simulink model "PID_mgtXY_loadingTest_video"  (R2023a)
settings: Solver=VariableStepAuto  StartTime=0.0  StopTime=t_sim/10  RelTol=1e-3
undefined symbols (not defined in the file or in its folder): A, B, DeltaH_error_Gain, Error_ref_Gain, I, J, juliandate, Ke, Kt, La, magnetic_field, Mgt_power_Gain, n_cal, omegaZ_inicial, R_mgt, Ra, RW_omega_max, RW_power_Gain, T_ext, T_max, T_max_mgt, yaw_ref
libraries: slpidlib x12, matrix_library x10, simulink_extras x6, sharedutil x3, simulink x2, vrlib x2, aerolibutil x1, sharedtransform x1, aerolibcubesatveh x1, aerolibgravity2 x1
(part 1 of 2)
settings Model: Creator=Personal  LastModifiedBy=Personal
settings SolverCC: ZeroCrossAlgorithm=Adaptive
settings DebuggingCC: IgnoredZcDiagnostic=none

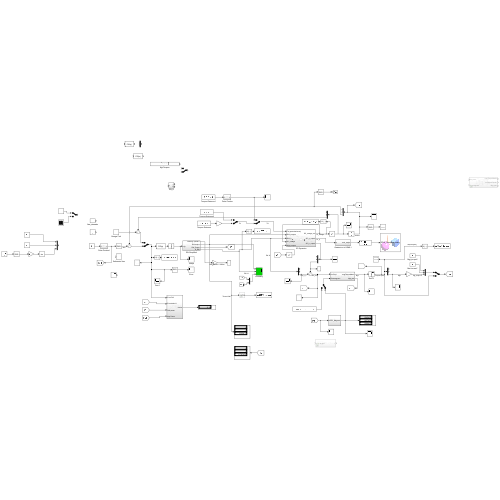
[thumbnail: Simulink's stored preview of the top-level diagram]
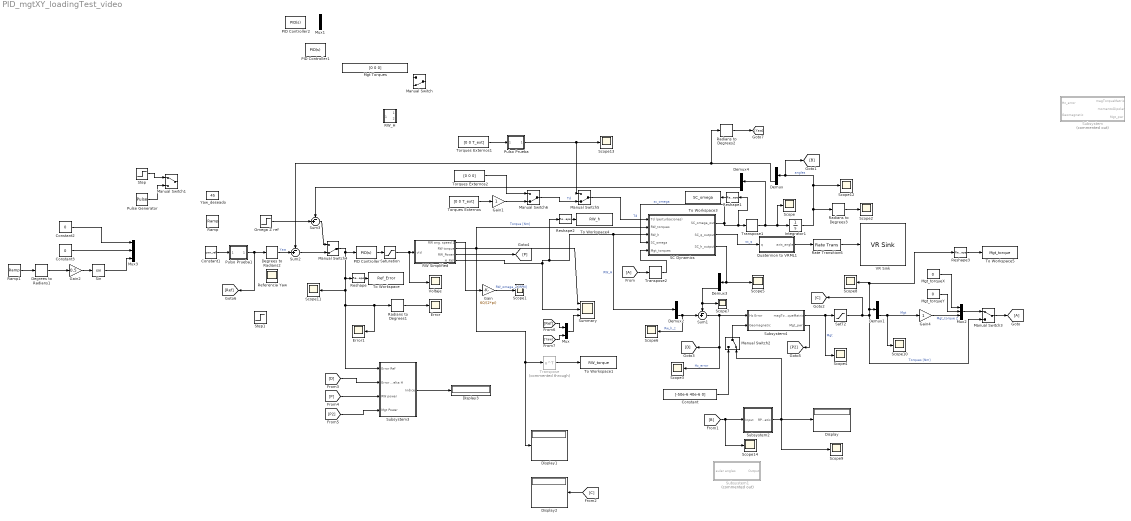
== system PID_mgtXY_loadingTest_video ==
  Constant : Constant  Value=[-50e-6 40e-6 0]
  Constant1 : Constant  Value=yaw_ref
  Constant2 : Constant  Value=0
  Constant3 : Constant  Value=0
  Degrees to Radians1 : simulink_extras/Transformations/Degrees to Radians
  Degrees to Radians2 : simulink_extras/Transformations/Degrees to Radians
  Demux{,1..4} (5 alike) : Demux  Outputs=3
  Display{,1..3} (4 alike) : Display
  Error : Scope
  Error1 : Scope
  From : From
  Gain : Gain  Gain=60/(2*pi)
  Gain1 : Gain
  Gain2 : Gain  Gain=0.5
  Gain4 : Gain
  Goto : Goto
  Integrator1 : Integrator  InitialCondition=[0 0 0]
  Manual Switch{,2,4..6} (5 alike) : ManualSwitch  CurrentSetting=0
  Manual Switch1 : ManualSwitch
  Manual Switch3 : ManualSwitch
  Mgt Torques : Constant  Value=[0 0 0]
  Mgt_torqueX : Constant  Value=0
  Mgt_torqueY : Constant  Value=0
  Mux : Mux  Inputs=2
  Mux1 : Mux  Inputs=3
  Mux2 : Mux  Inputs=3
  Mux3 : Mux  Inputs=3
  Omega Z ref : Step  Time=5  After=0.05  SampleTime=0
  PID Controller : slpidlib/PID Controller  Controller=PID  Form=Parallel  TimeDomain=Continuous-time  UseExternalTs=off  SampleTime=-1  IntegratorMethod=Forward Euler  FilterMethod=Forward Euler  ControllerParametersSource=internal  P=4500  I=800  UseKiTs=off  D=8000  N=100  UseFilter=on  TunerSelectOption=Transfer Function Based (PID Tuner App)  InitialConditionSource=internal  InitialConditionForIntegrator=0  InitialConditionForFilter=0  DifferentiatorICPrevScaledInput=0  ExternalReset=none  TrackingMode=off  Kt=1  LimitOutput=off  SatLimitsSource=internal  UpperSaturationLimit=1  LowerSaturationLimit=-1  LinearizeAsGain=on  AntiWindupMode=none  Kb=1  LimitIntegrator=off  UpperIntegratorSaturationLimit=inf  LowerIntegratorSaturationLimit=-inf  POutMin=[]  POutMax=[]  IOutMin=[]  IOutMax=[]  DOutMin=[]  DOutMax=[]  NOutMin=[]  NOutMax=[]  SumOutMin=[]  SumOutMax=[]  SaturationOutMin=[]  SaturationOutMax=[]  PParamMin=[]  PParamMax=[]  IParamMin=[]  IParamMax=[]  DParamMin=[]  DParamMax=[]  NParamMin=[]  NParamMax=[]  KbParamMin=[]  KbParamMax=[]  KtParamMin=[]  KtParamMax=[]  KbOutMin=[]  KbOutMax=[]  KtOutMin=[]  KtOutMax=[]  IntegratorOutMin=[]  IntegratorOutMax=[]  FilterOutMin=[]  FilterOutMax=[]  SumI1OutMin=[]  SumI1OutMax=[]  SumI2OutMin=[]  SumI2OutMax=[]  SumI3OutMin=[]  SumI3OutMax=[]  SumI4OutMin=[]  SumI4OutMax=[]  SumDOutMin=[]  SumDOutMax=[]  DifferentiatorOutMin=[]  DifferentiatorOutMax=[]  FilterDiffOutCoefMin=[]  FilterDiffOutCoefMax=[]  ReciprocalOutMin=[]  ReciprocalOutMax=[]  SumDenOutMin=[]  SumDenOutMax=[]  SumNumOutMin=[]  SumNumOutMax=[]  DivideOutMin=[]  DivideOutMax=[]  UdiffTsProdOutMin=[]  UdiffTsProdOutMax=[]  NTsProdOutMin=[]  NTsProdOutMax=[]  UintegralTsProdOutMin=[]  UintegralTsProdOutMax=[]  UngainTsProdOutMin=[]  UngainTsProdOutMax=[]  ClampingZeroOutDataTypeStr=Inherit: Inherit via back propagation  ClampingZeroOutMin=[]  ClampingZeroOutMax=[]  FilterDenConstantOutDataTypeStr=Inherit: Inherit via back propagation  FilterDenConstantOutMin=[]  FilterDenConstantOutMax=[]  PCopyOutDataTypeStr=Inherit: Inherit via back propagation  PCopyOutMin=[]  PCopyOutMax=[]  NCopyOutDataTypeStr=Inherit: Inherit via back propagation  NCopyOutMin=[]  NCopyOutMax=[]  IntegratorContinuousStateAttributes=''  IntegratorStateMustResolveToSignalObject=off  IntegratorRTWStateStorageClass=Auto  FilterContinuousStateAttributes=''  FilterStateMustResolveToSignalObject=off  FilterRTWStateStorageClass=Auto  ParallelPVariant=InternalParameters  IdealPVariant=Disabled  IVariant=InternalParameters  DVariant=InternalParameters  IntegratorVariant=Continuous  SatVariant=Disabled  AWVariant=Passthrough  PCopyVariant=Disabled  TRVariant=Disabled  FdbkBlocksVariant=Forward  IdealPFdbkVariant=Disabled  SatFdbkVariant=Disabled  DerivativeFilterVariant=ContFilter  NVariant=InternalParameters  NCopyVariant=Disabled  FilterICVariant=InternalICsFilter  IntegratorICVariant=InternalICs  ExternalResetVariant=Disabled  TRSumVariant=Passthrough  SumFdbkVariant=Disabled  SumVariant=Sum_PID  TsampFilterVariant=InternalTs  TsampNgainVariant=Passthrough  TsampIntegralVariant=Disabled_SignalSpec  ExternalSaturationOutDataTypeStr=Inherit: Same as second input
  PID Controller1 : slpidlib/PID Controller  Controller=PID  Form=Parallel  TimeDomain=Continuous-time  UseExternalTs=off  SampleTime=-1  IntegratorMethod=Forward Euler  FilterMethod=Forward Euler  ControllerParametersSource=internal  P=450  I=800  UseKiTs=off  D=8000  N=100  UseFilter=on  TunerSelectOption=Transfer Function Based (PID Tuner App)  InitialConditionSource=internal  InitialConditionForIntegrator=0  InitialConditionForFilter=0  DifferentiatorICPrevScaledInput=0  ExternalReset=none  TrackingMode=off  Kt=1  LimitOutput=off  SatLimitsSource=internal  UpperSaturationLimit=1  LowerSaturationLimit=-1  LinearizeAsGain=on  AntiWindupMode=none  Kb=1  LimitIntegrator=off  UpperIntegratorSaturationLimit=inf  LowerIntegratorSaturationLimit=-inf  POutMin=[]  POutMax=[]  IOutMin=[]  IOutMax=[]  DOutMin=[]  DOutMax=[]  NOutMin=[]  NOutMax=[]  SumOutMin=[]  SumOutMax=[]  SaturationOutMin=[]  SaturationOutMax=[]  PParamMin=[]  PParamMax=[]  IParamMin=[]  IParamMax=[]  DParamMin=[]  DParamMax=[]  NParamMin=[]  NParamMax=[]  KbParamMin=[]  KbParamMax=[]  KtParamMin=[]  KtParamMax=[]  KbOutMin=[]  KbOutMax=[]  KtOutMin=[]  KtOutMax=[]  IntegratorOutMin=[]  IntegratorOutMax=[]  FilterOutMin=[]  FilterOutMax=[]  SumI1OutMin=[]  SumI1OutMax=[]  SumI2OutMin=[]  SumI2OutMax=[]  SumI3OutMin=[]  SumI3OutMax=[]  SumI4OutMin=[]  SumI4OutMax=[]  SumDOutMin=[]  SumDOutMax=[]  DifferentiatorOutMin=[]  DifferentiatorOutMax=[]  FilterDiffOutCoefMin=[]  FilterDiffOutCoefMax=[]  ReciprocalOutMin=[]  ReciprocalOutMax=[]  SumDenOutMin=[]  SumDenOutMax=[]  SumNumOutMin=[]  SumNumOutMax=[]  DivideOutMin=[]  DivideOutMax=[]  UdiffTsProdOutMin=[]  UdiffTsProdOutMax=[]  NTsProdOutMin=[]  NTsProdOutMax=[]  UintegralTsProdOutMin=[]  UintegralTsProdOutMax=[]  UngainTsProdOutMin=[]  UngainTsProdOutMax=[]  ClampingZeroOutDataTypeStr=Inherit: Inherit via back propagation  ClampingZeroOutMin=[]  ClampingZeroOutMax=[]  FilterDenConstantOutDataTypeStr=Inherit: Inherit via back propagation  FilterDenConstantOutMin=[]  FilterDenConstantOutMax=[]  PCopyOutDataTypeStr=Inherit: Inherit via back propagation  PCopyOutMin=[]  PCopyOutMax=[]  NCopyOutDataTypeStr=Inherit: Inherit via back propagation  NCopyOutMin=[]  NCopyOutMax=[]  IntegratorContinuousStateAttributes=''  IntegratorStateMustResolveToSignalObject=off  IntegratorRTWStateStorageClass=Auto  FilterContinuousStateAttributes=''  FilterStateMustResolveToSignalObject=off  FilterRTWStateStorageClass=Auto  ParallelPVariant=InternalParameters  IdealPVariant=Disabled  IVariant=InternalParameters  DVariant=InternalParameters  IntegratorVariant=Continuous  SatVariant=Disabled  AWVariant=Passthrough  PCopyVariant=Disabled  TRVariant=Disabled  FdbkBlocksVariant=Forward  IdealPFdbkVariant=Disabled  SatFdbkVariant=Disabled  DerivativeFilterVariant=ContFilter  NVariant=InternalParameters  NCopyVariant=Disabled  FilterICVariant=InternalICsFilter  IntegratorICVariant=InternalICs  ExternalResetVariant=Disabled  TRSumVariant=Passthrough  SumFdbkVariant=Disabled  SumVariant=Sum_PID  TsampFilterVariant=InternalTs  TsampNgainVariant=Passthrough  TsampIntegralVariant=Disabled_SignalSpec  ExternalSaturationOutDataTypeStr=Inherit: Same as second input
  PID Controller2 : slpidlib/PID Controller  Controller=PID  Form=Parallel  TimeDomain=Continuous-time  UseExternalTs=off  SampleTime=-1  IntegratorMethod=Forward Euler  FilterMethod=Forward Euler  ControllerParametersSource=internal  P=4500  I=800  UseKiTs=off  D=8000  N=100  UseFilter=on  TunerSelectOption=Transfer Function Based (PID Tuner App)  InitialConditionSource=internal  InitialConditionForIntegrator=0  InitialConditionForFilter=0  DifferentiatorICPrevScaledInput=0  ExternalReset=none  TrackingMode=off  Kt=1  LimitOutput=off  SatLimitsSource=internal  UpperSaturationLimit=1  LowerSaturationLimit=-1  LinearizeAsGain=on  AntiWindupMode=none  Kb=1  LimitIntegrator=off  UpperIntegratorSaturationLimit=inf  LowerIntegratorSaturationLimit=-inf  POutMin=[]  POutMax=[]  IOutMin=[]  IOutMax=[]  DOutMin=[]  DOutMax=[]  NOutMin=[]  NOutMax=[]  SumOutMin=[]  SumOutMax=[]  SaturationOutMin=[]  SaturationOutMax=[]  PParamMin=[]  PParamMax=[]  IParamMin=[]  IParamMax=[]  DParamMin=[]  DParamMax=[]  NParamMin=[]  NParamMax=[]  KbParamMin=[]  KbParamMax=[]  KtParamMin=[]  KtParamMax=[]  KbOutMin=[]  KbOutMax=[]  KtOutMin=[]  KtOutMax=[]  IntegratorOutMin=[]  IntegratorOutMax=[]  FilterOutMin=[]  FilterOutMax=[]  SumI1OutMin=[]  SumI1OutMax=[]  SumI2OutMin=[]  SumI2OutMax=[]  SumI3OutMin=[]  SumI3OutMax=[]  SumI4OutMin=[]  SumI4OutMax=[]  SumDOutMin=[]  SumDOutMax=[]  DifferentiatorOutMin=[]  DifferentiatorOutMax=[]  FilterDiffOutCoefMin=[]  FilterDiffOutCoefMax=[]  ReciprocalOutMin=[]  ReciprocalOutMax=[]  SumDenOutMin=[]  SumDenOutMax=[]  SumNumOutMin=[]  SumNumOutMax=[]  DivideOutMin=[]  DivideOutMax=[]  UdiffTsProdOutMin=[]  UdiffTsProdOutMax=[]  NTsProdOutMin=[]  NTsProdOutMax=[]  UintegralTsProdOutMin=[]  UintegralTsProdOutMax=[]  UngainTsProdOutMin=[]  UngainTsProdOutMax=[]  ClampingZeroOutDataTypeStr=Inherit: Inherit via back propagation  ClampingZeroOutMin=[]  ClampingZeroOutMax=[]  FilterDenConstantOutDataTypeStr=Inherit: Inherit via back propagation  FilterDenConstantOutMin=[]  FilterDenConstantOutMax=[]  PCopyOutDataTypeStr=Inherit: Inherit via back propagation  PCopyOutMin=[]  PCopyOutMax=[]  NCopyOutDataTypeStr=Inherit: Inherit via back propagation  NCopyOutMin=[]  NCopyOutMax=[]  IntegratorContinuousStateAttributes=''  IntegratorStateMustResolveToSignalObject=off  IntegratorRTWStateStorageClass=Auto  FilterContinuousStateAttributes=''  FilterStateMustResolveToSignalObject=off  FilterRTWStateStorageClass=Auto  ParallelPVariant=InternalParameters  IdealPVariant=Disabled  IVariant=InternalParameters  DVariant=InternalParameters  IntegratorVariant=Continuous  SatVariant=Disabled  AWVariant=Passthrough  PCopyVariant=Disabled  TRVariant=Disabled  FdbkBlocksVariant=Forward  IdealPFdbkVariant=Disabled  SatFdbkVariant=Disabled  DerivativeFilterVariant=ContFilter  NVariant=InternalParameters  NCopyVariant=Disabled  FilterICVariant=InternalICsFilter  IntegratorICVariant=InternalICs  ExternalResetVariant=Disabled  TRSumVariant=Passthrough  SumFdbkVariant=Disabled  SumVariant=Sum_PID  TsampFilterVariant=InternalTs  TsampNgainVariant=Passthrough  TsampIntegralVariant=Disabled_SignalSpec  ExternalSaturationOutDataTypeStr=Inherit: Same as second input
  Pulse Generator : DiscretePulseGenerator  PulseType=Time based  Amplitude=45  Period=50  PulseWidth=50
  Pulso Prueba : Subsystem
  Pulso Prueba1 : Subsystem
  Quaternion to VRML1 : Subsystem
  RW Simplified : Subsystem
  RW_H : Subsystem
  Radians to Degrees1 : simulink_extras/Transformations/Radians to Degrees
  Radians to Degrees2 : simulink_extras/Transformations/Radians to Degrees
  Radians to Degrees3 : simulink_extras/Transformations/Radians to Degrees
  Ramp : simulink/Sources/Ramp  slope=1  start=0  InitialOutput=0
  Ramp1 : simulink/Sources/Ramp  slope=0.5  start=0  InitialOutput=0
  Rate Transition6 : RateTransition
  Referencia Yaw : Scope
  Reshape{,1..3} (4 alike) : Reshape
  SC Dynamics : Subsystem
  SatT2 : Saturate  UpperLimit=T_max_mgt  LowerLimit=-T_max_mgt
  Saturation : Saturate  UpperLimit=6  LowerLimit=-6
  Scope{,1..14} (15 alike) : Scope
  Sin : Trigonometry
  Step : Step  Time=5  After=60  SampleTime=0
  Step1 : Step  Time=0  SampleTime=0
  Subsystem : Subsystem  Commented=on
  Subsystem1 : Subsystem  Commented=on
  Subsystem2 : Subsystem
  Subsystem3 : Subsystem
  Subsystem4 : Subsystem
  Sum1 : Sum  Inputs=-+|
  Sum2 : Sum  Inputs=-+|
  Sum3 : Sum  Inputs=-+|
  Summary : Scope  NumInputPorts=3
  To Workspace : ToWorkspace  VariableName=Ref_Error  SaveFormat=Structure With Time  SampleTime=-1
  To Workspace1 : ToWorkspace  VariableName=RW_torque  SaveFormat=Structure With Time  SampleTime=-1
  To Workspace3 : ToWorkspace  VariableName=SC_omega  SaveFormat=Structure With Time  SampleTime=-1
  To Workspace4 : ToWorkspace  VariableName=RW_h  SaveFormat=Structure With Time  SampleTime=-1
  To Workspace5 : ToWorkspace  VariableName=Mgt_torque  SaveFormat=Structure With Time  SampleTime=-1
  Torques Externos : Constant  Value=[0 0 T_ext]
  Torques Externos1 : Constant  Value=[0 0 T_ext]
  Torques Externos2 : Constant  Value=[0 0 0]
  Transpose : Math  Commented=through  Operator=transpose
  Transpose1 : matrix_library/Transpose
  Transpose2 : matrix_library/Transpose
  VR Sink : vrlib/VR Sink  InstantiateOnLoad=on  SampleTime=0.1  ViewEnable=on  RemoteChange=off  RemoteView=off  FieldsWritten=STLB_Transform.rotation.4.1.1.double  WorldFileName=EscenarioCubeSat.x3d  AutoView=off  VideoDimensions=[]  AllowVariableSize=off
  Voltaje : Scope
  Yaw_deseado : Constant  Value=45
  wires:
  Torques Externos/1 -> Gain1/1
  SC Dynamics/1(SC_omega_out) -> Reshape1/1, Transpose1/1, SC Dynamics/4(SC_omega)  "sc_omega"
  Integrator1/1 -> Radians to Degrees3/1, Scope12/1, [B], Demux/1  "angles"
  Demux/3 -> Radians to Degrees2/1, Sum2/1
  Saturation/1 -> Voltaje/1, RW Simplified/1(v(t))
  Transpose1/1 -> Demux4/1, Scope/1, Integrator1/1
  RW Simplified/2(RW torque) -> SC Dynamics/2(RW_torques), Transpose/1, Display1/1, Summary/1  "Torque [Nm]"
  SC Dynamics/2(SC_q_output) -> Quaternion to VRML1/1(q)  "sc_q"
  Quaternion to VRML1/1(axis_angle) -> Rate Transition6/1
  Rate Transition6/1 -> VR Sink/1
  Radians to Degrees1/1 -> Error/1
  Radians to Degrees3/1 -> Scope2/1
  Gain/1 -> Scope1/1  "RW_omega_Z [RPM]"
  Manual Switch5/1 -> SC Dynamics/1(Td (perturbaciones))  "Td"
  SC Dynamics/3(SC_h_output) -> Scope5/1, Demux3/1
  Demux2/3 -> Scope6/1, Sum1/2  "Rw_h_z"
  Demux3/3 -> Sum1/1, Scope7/1
  Mgt_torqueX/1 -> Mux2/1
  Mgt_torqueY/1 -> Mux2/2
  Gain4/1 -> Mux2/3  "Mgt_torque Z"
  RW Simplified/4(H_RW) -> Reshape2/1, Demux2/1, SC Dynamics/3(RW_h), Summary/2  "RW_H"
  RW Simplified/1(RW ang. speed Z) -> Gain/1
  PID Controller/1 -> Saturation/1
  From/1 -> Transpose2/1
  Pulse Generator/1 -> Manual Switch1/2
  Step/1 -> Manual Switch1/1
  Demux1/3 -> Scope10/1, Gain4/1  "Mgt"
  Sum1/1 -> [D], Scope3/1, Subsystem4/1(Hz Error)  "Hz_error"
  Constant/1 -> Manual Switch2/1
  Manual Switch2/1 -> Subsystem4/2(Geomagnetic)
  Subsystem2/1(RPY_Magnetic) -> Display/1, Scope9/1, Manual Switch2/2
  [B] -> Scope14/1, Subsystem2/1(Input)
  Transpose2/1 -> SC Dynamics/5(Mgt_torques)
  Manual Switch3/1 -> Goto/1
  Mux2/1 -> Manual Switch3/1
  [C] -> Display2/1
  Demux4/3 -> Sum3/1
  Omega Z ref/1 -> Sum3/2
  Sum2/1 -> Manual Switch4/2
  Sum3/1 -> Manual Switch4/1
  RW Simplified/3(RW_Power) -> [P]
  [D] -> Subsystem3/2(Error delta H)
  [P] -> Subsystem3/3(RW power)
  [P2] -> Subsystem3/4(Mgt Power)
  Subsystem3/1(Indice) -> Display3/1
  Subsystem4/1(magTorqueMatrix) -> Scope4/1, SatT2/1  "Mgt"
  Subsystem4/2(Mgt_pwr) -> [P2]
  Pulso Prueba/1(Out1) -> Scope13/1, Manual Switch5/1
  Torques Externos1/1 -> Pulso Prueba/1(In1)
  Constant1/1 -> Pulso Prueba1/1(In1)
  Torques Externos2/1 -> Manual Switch6/1
  Manual Switch6/1 -> Manual Switch5/2  "Td"
  Gain1/1 -> Manual Switch6/2
  [Ref] -> Mux/1
  [Yaw] -> Mux/2
  Mux/1 -> Summary/3
  Transpose/1 -> To Workspace1/1
  Manual Switch4/1 -> PID Controller/1, Scope11/1, Subsystem3/1(Error Ref), Error1/1, Radians to Degrees1/1, Reshape/1
  Reshape/1 -> To Workspace/1
  Constant3/1 -> Mux3/2
  Constant2/1 -> Mux3/1
  Sin/1 -> Mux3/3
  Degrees to Radians1/1 -> Gain2/1
  Gain2/1 -> Sin/1
  Ramp1/1 -> Degrees to Radians1/1
  Radians to Degrees2/1 -> [Yaw]
  Pulso Prueba1/1(Out1) -> [Ref], Degrees to Radians2/1
  Degrees to Radians2/1 -> Sum2/2  "Yaw"
  Reshape1/1 -> To Workspace3/1
  Reshape2/1 -> To Workspace4/1
  SatT2/1 -> [C], Manual Switch3/2, Demux1/1, Reshape3/1, Scope8/1  "Torques [Nm]"
  Reshape3/1 -> To Workspace5/1

== system PID_mgtXY_loadingTest_video/Pulso Prueba ==
  In1 : Inport
  Product1 : Product
  Scope5 : Scope
  Step2 : Step  Time=500  SampleTime=0
  Step3 : Step  Time=6000  After=-2  SampleTime=0
  Sum : Sum  Inputs=|++
  Out1 : Outport
  wires:
  Step2/1 -> Sum/1
  Step3/1 -> Sum/2
  In1/1 -> Product1/2
  Sum/1 -> Product1/1, Scope5/1
  Product1/1 -> Out1/1

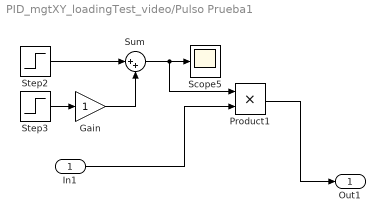
== system PID_mgtXY_loadingTest_video/Pulso Prueba1 ==
  In1 : Inport
  Gain : Gain
  Product1 : Product
  Scope5 : Scope
  Step2 : Step  Time=15  SampleTime=0
  Step3 : Step  Time=50  SampleTime=0
  Sum : Sum  Inputs=|++
  Out1 : Outport
  wires:
  Product1/1 -> Out1/1
  Sum/1 -> Scope5/1, Product1/1
  In1/1 -> Product1/2
  Step3/1 -> Gain/1
  Step2/1 -> Sum/1
  Gain/1 -> Sum/2

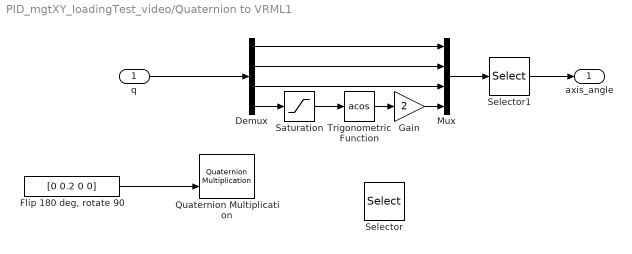
== system PID_mgtXY_loadingTest_video/Quaternion to VRML1 ==
  q : Inport
  Demux : Demux
  "Flip 180 deg, rotate 90" : Constant  Value=[0 0.2 0 0]
  Gain : Gain  Gain=2
  Mux : Mux
  Quaternion Multiplication : aerolibutil/Quaternion Multiplication
  Saturation : Saturate  UpperLimit=1  LowerLimit=-1  ZeroCross=off
  Selector : Selector  InputPortWidth=3  IndexOptions=Index vector (dialog)  Indices=[1 3]  OutputSizes=1
  Selector1 : Selector  InputPortWidth=4  IndexOptions=Index vector (dialog)  Indices=[2 3 1 4]  OutputSizes=1
  Trigonometric Function : Trigonometry  Operator=acos
  axis_angle : Outport  VectorParamsAs1DForOutWhenUnconnected=off
  wires:
  Demux/2 -> Mux/2
  "Flip 180 deg, rotate 90"/1 -> Quaternion Multiplication/2
  q/1 -> Demux/1
  Demux/1 -> Mux/1
  Mux/1 -> Selector1/1
  Selector1/1 -> axis_angle/1
  Trigonometric Function/1 -> Gain/1
  Gain/1 -> Mux/4
  Demux/3 -> Mux/3
  Saturation/1 -> Trigonometric Function/1
  Demux/4 -> Saturation/1

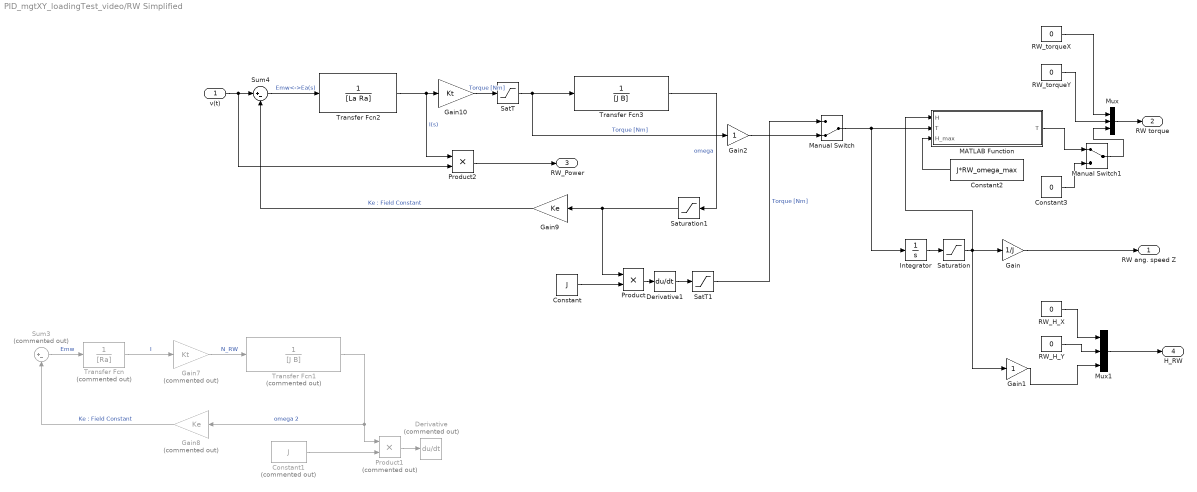
== system PID_mgtXY_loadingTest_video/RW Simplified ==
  v(t) : Inport
  Constant : Constant  Value=J
  Constant1 : Constant  Commented=on  Value=J
  Constant2 : Constant  Value=J*RW_omega_max
  Constant3 : Constant  Value=0
  Derivative : Derivative  Commented=on
  Derivative1 : Derivative
  Gain : Gain  Gain=1/J
  Gain1 : Gain
  Gain10 : Gain  Gain=Kt
  Gain2 : Gain
  Gain7 : Gain  Commented=on  Gain=Kt
  Gain8 : Gain  Commented=on  Gain=Ke
  Gain9 : Gain  Gain=Ke
  Integrator : Integrator
  MATLAB Function : MATLAB Function  TreatAsAtomicUnit=on
  Manual Switch : ManualSwitch  CurrentSetting=0
  Manual Switch1 : ManualSwitch
  Mux : Mux  Inputs=3
  Mux1 : Mux  Inputs=3
  Product : Product
  Product1 : Product  Commented=on
  Product2 : Product
  RW_H_X : Constant  Value=0
  RW_H_Y : Constant  Value=0
  RW_torqueX : Constant  Value=0
  RW_torqueY : Constant  Value=0
  SatT : Saturate  UpperLimit=T_max  LowerLimit=-T_max
  SatT1 : Saturate  UpperLimit=T_max  LowerLimit=-T_max
  Saturation : Saturate  UpperLimit=J*RW_omega_max  LowerLimit=-J*RW_omega_max
  Saturation1 : Saturate  UpperLimit=RW_omega_max  LowerLimit=-RW_omega_max
  Sum3 : Sum  Commented=on  Inputs=|+-
  Sum4 : Sum  Inputs=|+-
  Transfer Fcn : TransferFcn  Commented=on  Denominator=[Ra]
  Transfer Fcn1 : TransferFcn  Commented=on  Denominator=[J B]
  Transfer Fcn2 : TransferFcn  Denominator=[La Ra]
  Transfer Fcn3 : TransferFcn  Denominator=[J B]
  RW ang. speed Z : Outport  VectorParamsAs1DForOutWhenUnconnected=off
  RW torque : Outport  Port=2  VectorParamsAs1DForOutWhenUnconnected=off
  RW_Power : Outport  Port=3  VectorParamsAs1DForOutWhenUnconnected=off
  H_RW : Outport  Port=4  VectorParamsAs1DForOutWhenUnconnected=off
  wires:
  Transfer Fcn2/1 -> Product2/1, Gain10/1  "I(s)"
  Sum4/1 -> Transfer Fcn2/1  "Emw<->Ea(s)"
  Gain9/1 -> Sum4/2  "Ke : Field Constant"
  Transfer Fcn3/1 -> Saturation1/1  "omega"
  Constant/1 -> Product/2
  Integrator/1 -> Saturation/1
  v(t)/1 -> Product2/2, Sum4/1
  Product1/1 -> Derivative/1
  Constant1/1 -> Product1/2
  Transfer Fcn1/1 -> Product1/1, Gain8/1  "omega 2"
  Gain7/1 -> Transfer Fcn1/1  "N_RW"
  Sum3/1 -> Transfer Fcn/1  "Emw"
  Transfer Fcn/1 -> Gain7/1  "I"
  Gain8/1 -> Sum3/2  "Ke : Field Constant"
  RW_H_X/1 -> Mux1/1
  RW_H_Y/1 -> Mux1/2
  Mux1/1 -> H_RW/1
  RW_torqueX/1 -> Mux/1
  RW_torqueY/1 -> Mux/2
  Mux/1 -> RW torque/1
  Gain10/1 -> SatT/1  "Torque [Nm]"
  SatT/1 -> Gain2/1, Transfer Fcn3/1  "Torque [Nm]"
  Gain/1 -> RW ang. speed Z/1
  Gain1/1 -> Mux1/3
  Product2/1 -> RW_Power/1
  Saturation/1 -> Gain/1, Gain1/1, MATLAB Function/1(H)
  Product/1 -> Derivative1/1
  Derivative1/1 -> SatT1/1
  SatT1/1 -> Manual Switch/1  "Torque [Nm]"
  Manual Switch/1 -> Integrator/1, MATLAB Function/2("T ")
  Saturation1/1 -> Gain9/1, Product/1
  Constant2/1 -> MATLAB Function/3(H_max)
  Manual Switch1/1 -> Mux/3
  Gain2/1 -> Manual Switch/2
  MATLAB Function/1(T) -> Manual Switch1/1
  Constant3/1 -> Manual Switch1/2

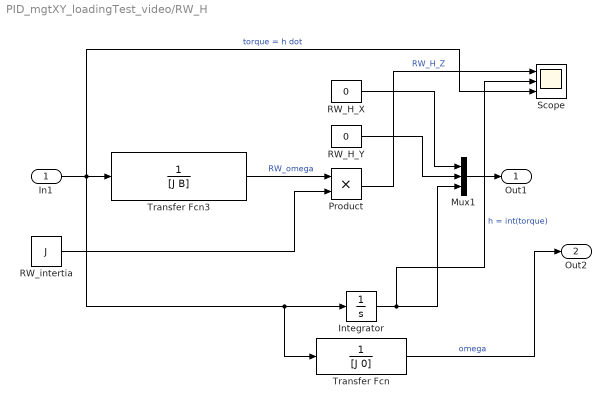
== system PID_mgtXY_loadingTest_video/RW_H ==
  In1 : Inport
  Integrator : Integrator
  Mux1 : Mux  Inputs=3
  Product : Product
  RW_H_X : Constant  Value=0
  RW_H_Y : Constant  Value=0
  RW_intertia : Constant  Value=J
  Scope : Scope  NumInputPorts=3
  Transfer Fcn : TransferFcn  Denominator=[J 0]
  Transfer Fcn3 : TransferFcn  Denominator=[J B]
  Out1 : Outport
  Out2 : Outport  Port=2
  wires:
  RW_H_Y/1 -> Mux1/2
  RW_intertia/1 -> Product/2
  In1/1 -> Scope/3, Transfer Fcn3/1, Transfer Fcn/1, Integrator/1  "torque = h dot"
  RW_H_X/1 -> Mux1/1
  Mux1/1 -> Out1/1
  Transfer Fcn3/1 -> Product/1  "RW_omega"
  Integrator/1 -> Scope/2, Mux1/3  "h = int(torque)"
  Transfer Fcn/1 -> Out2/1  "omega"
  Product/1 -> Scope/1  "RW_H_Z"

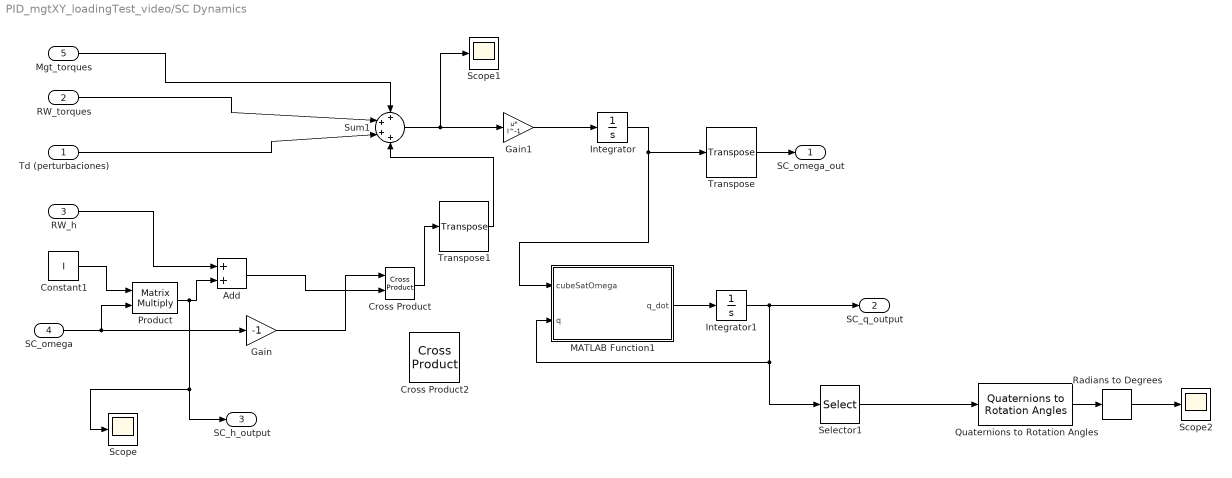
== system PID_mgtXY_loadingTest_video/SC Dynamics ==
  Td (perturbaciones) : Inport
  RW_torques : Inport  Port=2
  RW_h : Inport  Port=3
  SC_omega : Inport  Port=4
  Mgt_torques : Inport  Port=5
  Add : Sum
  Constant1 : Constant  Value=I
  Cross Product : vrlib/Utilities/Cross Product
  Cross Product2 : matrix_library/Cross Product
  Gain : Gain  Gain=-1
  Gain1 : Gain  Gain=I^-1  Multiplication=Matrix(u*K)
  Integrator : Integrator  InitialCondition=[0 0 omegaZ_inicial]
  Integrator1 : Integrator  InitialCondition=[0 0 0 1]
  MATLAB Function1 : MATLAB Function  TreatAsAtomicUnit=on
  Product : Product  Multiplication=Matrix(*)
  Quaternions to Rotation Angles : sharedtransform/Quaternions to Rotation Angles  rotationOrder=ZYX  aMode=aMode
  Radians to Degrees : simulink_extras/Transformations/Radians to Degrees
  Scope : Scope
  Scope1 : Scope
  Scope2 : Scope
  Selector1 : Selector  InputPortWidth=4  IndexOptions=Index vector (dialog)  Indices=[4 1 2 3]  OutputSizes=1
  Sum1 : Sum  Inputs=++++
  Transpose : matrix_library/Transpose
  Transpose1 : matrix_library/Transpose
  SC_omega_out : Outport
  SC_q_output : Outport  Port=2
  SC_h_output : Outport  Port=3
  wires:
  RW_torques/1 -> Sum1/2
  Td (perturbaciones)/1 -> Sum1/3
  Integrator1/1 -> Selector1/1, MATLAB Function1/2(q), SC_q_output/1
  Constant1/1 -> Product/1
  Product/1 -> Scope/1, SC_h_output/1, Add/2
  RW_h/1 -> Add/1
  Gain/1 -> Cross Product/1
  Add/1 -> Cross Product/2
  Cross Product/1 -> Transpose1/1
  Sum1/1 -> Scope1/1, Gain1/1
  Gain1/1 -> Integrator/1
  Integrator/1 -> MATLAB Function1/1(cubeSatOmega), Transpose/1
  MATLAB Function1/1(q_dot) -> Integrator1/1
  SC_omega/1 -> Product/2, Gain/1
  Transpose/1 -> SC_omega_out/1
  Transpose1/1 -> Sum1/4
  Mgt_torques/1 -> Sum1/1
  Quaternions to Rotation Angles/1 -> Radians to Degrees/1
  Radians to Degrees/1 -> Scope2/1
  Selector1/1 -> Quaternions to Rotation Angles/1

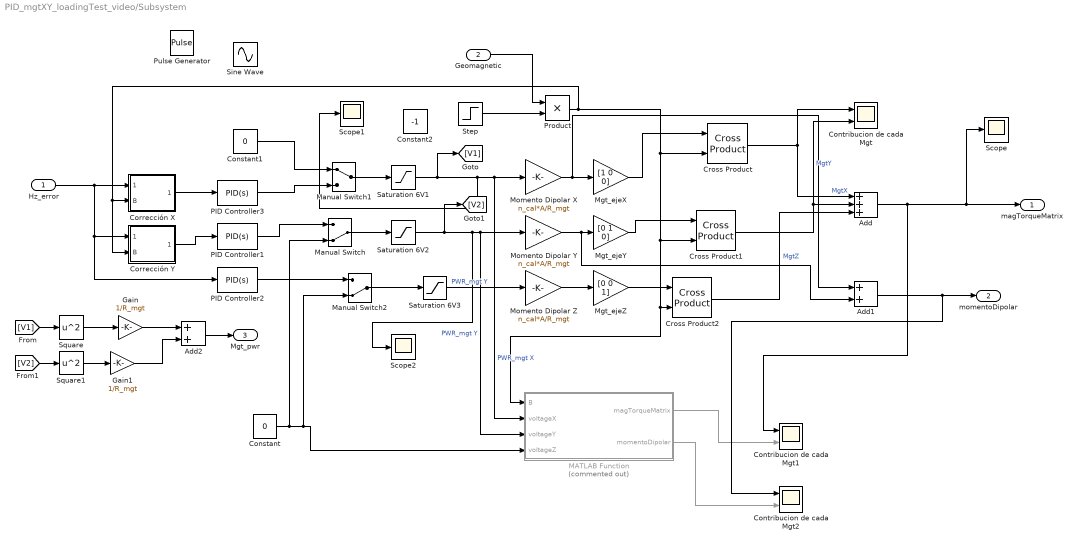
== system PID_mgtXY_loadingTest_video/Subsystem ==
  Hz_error : Inport
  Geomagnetic : Inport  Port=2
  Add : Sum  Inputs=+++
  Add1 : Sum
  Add2 : Sum
  Constant : Constant  Value=0
  Constant1 : Constant  Value=0
  Constant2 : Constant  Value=-1
  Contribucion de cada Mgt : Scope  NumInputPorts=2
  Contribucion de cada Mgt1 : Scope  NumInputPorts=2
  Contribucion de cada Mgt2 : Scope  NumInputPorts=2
  Corrección X : MATLAB Function  TreatAsAtomicUnit=on
  Corrección Y : MATLAB Function  TreatAsAtomicUnit=on
  Cross Product : matrix_library/Cross Product
  Cross Product1 : matrix_library/Cross Product
  Cross Product2 : matrix_library/Cross Product
  Gain : Gain  Gain=1/R_mgt
  Gain1 : Gain  Gain=1/R_mgt
  MATLAB Function : MATLAB Function  Commented=on  TreatAsAtomicUnit=on
  Manual Switch : ManualSwitch  CurrentSetting=0
  Manual Switch1 : ManualSwitch
  Manual Switch2 : ManualSwitch  CurrentSetting=0
  Mgt_ejeX : Gain  Gain=[1 0 0]
  Mgt_ejeY : Gain  Gain=[0 1 0]
  Mgt_ejeZ : Gain  Gain=[0 0 1]
  Momento Dipolar X : Gain  Gain=n_cal*A/R_mgt
  Momento Dipolar Y : Gain  Gain=n_cal*A/R_mgt
  Momento Dipolar Z : Gain  Gain=n_cal*A/R_mgt
  PID Controller1 : slpidlib/PID Controller  Controller=PID  Form=Parallel  TimeDomain=Continuous-time  UseExternalTs=off  SampleTime=-1  IntegratorMethod=Forward Euler  FilterMethod=Forward Euler  ControllerParametersSource=internal  P=4500  I=800  UseKiTs=off  D=8000  N=100  UseFilter=on  TunerSelectOption=Transfer Function Based (PID Tuner App)  InitialConditionSource=internal  InitialConditionForIntegrator=0  InitialConditionForFilter=0  DifferentiatorICPrevScaledInput=0  ExternalReset=none  TrackingMode=off  Kt=1  LimitOutput=off  SatLimitsSource=internal  UpperSaturationLimit=1  LowerSaturationLimit=-1  LinearizeAsGain=on  AntiWindupMode=none  Kb=1  LimitIntegrator=off  UpperIntegratorSaturationLimit=inf  LowerIntegratorSaturationLimit=-inf  POutMin=[]  POutMax=[]  IOutMin=[]  IOutMax=[]  DOutMin=[]  DOutMax=[]  NOutMin=[]  NOutMax=[]  SumOutMin=[]  SumOutMax=[]  SaturationOutMin=[]  SaturationOutMax=[]  PParamMin=[]  PParamMax=[]  IParamMin=[]  IParamMax=[]  DParamMin=[]  DParamMax=[]  NParamMin=[]  NParamMax=[]  KbParamMin=[]  KbParamMax=[]  KtParamMin=[]  KtParamMax=[]  KbOutMin=[]  KbOutMax=[]  KtOutMin=[]  KtOutMax=[]  IntegratorOutMin=[]  IntegratorOutMax=[]  FilterOutMin=[]  FilterOutMax=[]  SumI1OutMin=[]  SumI1OutMax=[]  SumI2OutMin=[]  SumI2OutMax=[]  SumI3OutMin=[]  SumI3OutMax=[]  SumI4OutMin=[]  SumI4OutMax=[]  SumDOutMin=[]  SumDOutMax=[]  DifferentiatorOutMin=[]  DifferentiatorOutMax=[]  FilterDiffOutCoefMin=[]  FilterDiffOutCoefMax=[]  ReciprocalOutMin=[]  ReciprocalOutMax=[]  SumDenOutMin=[]  SumDenOutMax=[]  SumNumOutMin=[]  SumNumOutMax=[]  DivideOutMin=[]  DivideOutMax=[]  UdiffTsProdOutMin=[]  UdiffTsProdOutMax=[]  NTsProdOutMin=[]  NTsProdOutMax=[]  UintegralTsProdOutMin=[]  UintegralTsProdOutMax=[]  UngainTsProdOutMin=[]  UngainTsProdOutMax=[]  ClampingZeroOutDataTypeStr=Inherit: Inherit via back propagation  ClampingZeroOutMin=[]  ClampingZeroOutMax=[]  FilterDenConstantOutDataTypeStr=Inherit: Inherit via back propagation  FilterDenConstantOutMin=[]  FilterDenConstantOutMax=[]  PCopyOutDataTypeStr=Inherit: Inherit via back propagation  PCopyOutMin=[]  PCopyOutMax=[]  NCopyOutDataTypeStr=Inherit: Inherit via back propagation  NCopyOutMin=[]  NCopyOutMax=[]  IntegratorContinuousStateAttributes=''  IntegratorStateMustResolveToSignalObject=off  IntegratorRTWStateStorageClass=Auto  FilterContinuousStateAttributes=''  FilterStateMustResolveToSignalObject=off  FilterRTWStateStorageClass=Auto  ParallelPVariant=InternalParameters  IdealPVariant=Disabled  IVariant=InternalParameters  DVariant=InternalParameters  IntegratorVariant=Continuous  SatVariant=Disabled  AWVariant=Passthrough  PCopyVariant=Disabled  TRVariant=Disabled  FdbkBlocksVariant=Forward  IdealPFdbkVariant=Disabled  SatFdbkVariant=Disabled  DerivativeFilterVariant=ContFilter  NVariant=InternalParameters  NCopyVariant=Disabled  FilterICVariant=InternalICsFilter  IntegratorICVariant=InternalICs  ExternalResetVariant=Disabled  TRSumVariant=Passthrough  SumFdbkVariant=Disabled  SumVariant=Sum_PID  TsampFilterVariant=InternalTs  TsampNgainVariant=Passthrough  TsampIntegralVariant=Disabled_SignalSpec  ExternalSaturationOutDataTypeStr=Inherit: Same as second input
  PID Controller2 : slpidlib/PID Controller  Controller=PID  Form=Parallel  TimeDomain=Continuous-time  UseExternalTs=off  SampleTime=-1  IntegratorMethod=Forward Euler  FilterMethod=Forward Euler  ControllerParametersSource=internal  P=4500  I=800  UseKiTs=off  D=8000  N=100  UseFilter=on  TunerSelectOption=Transfer Function Based (PID Tuner App)  InitialConditionSource=internal  InitialConditionForIntegrator=0  InitialConditionForFilter=0  DifferentiatorICPrevScaledInput=0  ExternalReset=none  TrackingMode=off  Kt=1  LimitOutput=off  SatLimitsSource=internal  UpperSaturationLimit=1  LowerSaturationLimit=-1  LinearizeAsGain=on  AntiWindupMode=none  Kb=1  LimitIntegrator=off  UpperIntegratorSaturationLimit=inf  LowerIntegratorSaturationLimit=-inf  POutMin=[]  POutMax=[]  IOutMin=[]  IOutMax=[]  DOutMin=[]  DOutMax=[]  NOutMin=[]  NOutMax=[]  SumOutMin=[]  SumOutMax=[]  SaturationOutMin=[]  SaturationOutMax=[]  PParamMin=[]  PParamMax=[]  IParamMin=[]  IParamMax=[]  DParamMin=[]  DParamMax=[]  NParamMin=[]  NParamMax=[]  KbParamMin=[]  KbParamMax=[]  KtParamMin=[]  KtParamMax=[]  KbOutMin=[]  KbOutMax=[]  KtOutMin=[]  KtOutMax=[]  IntegratorOutMin=[]  IntegratorOutMax=[]  FilterOutMin=[]  FilterOutMax=[]  SumI1OutMin=[]  SumI1OutMax=[]  SumI2OutMin=[]  SumI2OutMax=[]  SumI3OutMin=[]  SumI3OutMax=[]  SumI4OutMin=[]  SumI4OutMax=[]  SumDOutMin=[]  SumDOutMax=[]  DifferentiatorOutMin=[]  DifferentiatorOutMax=[]  FilterDiffOutCoefMin=[]  FilterDiffOutCoefMax=[]  ReciprocalOutMin=[]  ReciprocalOutMax=[]  SumDenOutMin=[]  SumDenOutMax=[]  SumNumOutMin=[]  SumNumOutMax=[]  DivideOutMin=[]  DivideOutMax=[]  UdiffTsProdOutMin=[]  UdiffTsProdOutMax=[]  NTsProdOutMin=[]  NTsProdOutMax=[]  UintegralTsProdOutMin=[]  UintegralTsProdOutMax=[]  UngainTsProdOutMin=[]  UngainTsProdOutMax=[]  ClampingZeroOutDataTypeStr=Inherit: Inherit via back propagation  ClampingZeroOutMin=[]  ClampingZeroOutMax=[]  FilterDenConstantOutDataTypeStr=Inherit: Inherit via back propagation  FilterDenConstantOutMin=[]  FilterDenConstantOutMax=[]  PCopyOutDataTypeStr=Inherit: Inherit via back propagation  PCopyOutMin=[]  PCopyOutMax=[]  NCopyOutDataTypeStr=Inherit: Inherit via back propagation  NCopyOutMin=[]  NCopyOutMax=[]  IntegratorContinuousStateAttributes=''  IntegratorStateMustResolveToSignalObject=off  IntegratorRTWStateStorageClass=Auto  FilterContinuousStateAttributes=''  FilterStateMustResolveToSignalObject=off  FilterRTWStateStorageClass=Auto  ParallelPVariant=InternalParameters  IdealPVariant=Disabled  IVariant=InternalParameters  DVariant=InternalParameters  IntegratorVariant=Continuous  SatVariant=Disabled  AWVariant=Passthrough  PCopyVariant=Disabled  TRVariant=Disabled  FdbkBlocksVariant=Forward  IdealPFdbkVariant=Disabled  SatFdbkVariant=Disabled  DerivativeFilterVariant=ContFilter  NVariant=InternalParameters  NCopyVariant=Disabled  FilterICVariant=InternalICsFilter  IntegratorICVariant=InternalICs  ExternalResetVariant=Disabled  TRSumVariant=Passthrough  SumFdbkVariant=Disabled  SumVariant=Sum_PID  TsampFilterVariant=InternalTs  TsampNgainVariant=Passthrough  TsampIntegralVariant=Disabled_SignalSpec  ExternalSaturationOutDataTypeStr=Inherit: Same as second input
  PID Controller3 : slpidlib/PID Controller  Controller=PID  Form=Parallel  TimeDomain=Continuous-time  UseExternalTs=off  SampleTime=-1  IntegratorMethod=Forward Euler  FilterMethod=Forward Euler  ControllerParametersSource=internal  P=4500  I=800  UseKiTs=off  D=8000  N=100  UseFilter=on  TunerSelectOption=Transfer Function Based (PID Tuner App)  InitialConditionSource=internal  InitialConditionForIntegrator=0  InitialConditionForFilter=0  DifferentiatorICPrevScaledInput=0  ExternalReset=none  TrackingMode=off  Kt=1  LimitOutput=off  SatLimitsSource=internal  UpperSaturationLimit=1  LowerSaturationLimit=-1  LinearizeAsGain=on  AntiWindupMode=none  Kb=1  LimitIntegrator=off  UpperIntegratorSaturationLimit=inf  LowerIntegratorSaturationLimit=-inf  POutMin=[]  POutMax=[]  IOutMin=[]  IOutMax=[]  DOutMin=[]  DOutMax=[]  NOutMin=[]  NOutMax=[]  SumOutMin=[]  SumOutMax=[]  SaturationOutMin=[]  SaturationOutMax=[]  PParamMin=[]  PParamMax=[]  IParamMin=[]  IParamMax=[]  DParamMin=[]  DParamMax=[]  NParamMin=[]  NParamMax=[]  KbParamMin=[]  KbParamMax=[]  KtParamMin=[]  KtParamMax=[]  KbOutMin=[]  KbOutMax=[]  KtOutMin=[]  KtOutMax=[]  IntegratorOutMin=[]  IntegratorOutMax=[]  FilterOutMin=[]  FilterOutMax=[]  SumI1OutMin=[]  SumI1OutMax=[]  SumI2OutMin=[]  SumI2OutMax=[]  SumI3OutMin=[]  SumI3OutMax=[]  SumI4OutMin=[]  SumI4OutMax=[]  SumDOutMin=[]  SumDOutMax=[]  DifferentiatorOutMin=[]  DifferentiatorOutMax=[]  FilterDiffOutCoefMin=[]  FilterDiffOutCoefMax=[]  ReciprocalOutMin=[]  ReciprocalOutMax=[]  SumDenOutMin=[]  SumDenOutMax=[]  SumNumOutMin=[]  SumNumOutMax=[]  DivideOutMin=[]  DivideOutMax=[]  UdiffTsProdOutMin=[]  UdiffTsProdOutMax=[]  NTsProdOutMin=[]  NTsProdOutMax=[]  UintegralTsProdOutMin=[]  UintegralTsProdOutMax=[]  UngainTsProdOutMin=[]  UngainTsProdOutMax=[]  ClampingZeroOutDataTypeStr=Inherit: Inherit via back propagation  ClampingZeroOutMin=[]  ClampingZeroOutMax=[]  FilterDenConstantOutDataTypeStr=Inherit: Inherit via back propagation  FilterDenConstantOutMin=[]  FilterDenConstantOutMax=[]  PCopyOutDataTypeStr=Inherit: Inherit via back propagation  PCopyOutMin=[]  PCopyOutMax=[]  NCopyOutDataTypeStr=Inherit: Inherit via back propagation  NCopyOutMin=[]  NCopyOutMax=[]  IntegratorContinuousStateAttributes=''  IntegratorStateMustResolveToSignalObject=off  IntegratorRTWStateStorageClass=Auto  FilterContinuousStateAttributes=''  FilterStateMustResolveToSignalObject=off  FilterRTWStateStorageClass=Auto  ParallelPVariant=InternalParameters  IdealPVariant=Disabled  IVariant=InternalParameters  DVariant=InternalParameters  IntegratorVariant=Continuous  SatVariant=Disabled  AWVariant=Passthrough  PCopyVariant=Disabled  TRVariant=Disabled  FdbkBlocksVariant=Forward  IdealPFdbkVariant=Disabled  SatFdbkVariant=Disabled  DerivativeFilterVariant=ContFilter  NVariant=InternalParameters  NCopyVariant=Disabled  FilterICVariant=InternalICsFilter  IntegratorICVariant=InternalICs  ExternalResetVariant=Disabled  TRSumVariant=Passthrough  SumFdbkVariant=Disabled  SumVariant=Sum_PID  TsampFilterVariant=InternalTs  TsampNgainVariant=Passthrough  TsampIntegralVariant=Disabled_SignalSpec  ExternalSaturationOutDataTypeStr=Inherit: Same as second input
  Product : Product
  Pulse Generator : DiscretePulseGenerator  PulseType=Time based  Period=80  PulseWidth=50  PhaseDelay=50
  Saturation 6V1 : Saturate  UpperLimit=5  LowerLimit=-5
  Saturation 6V2 : Saturate  UpperLimit=5  LowerLimit=-5
  Saturation 6V3 : Saturate  UpperLimit=5  LowerLimit=-5
  Scope : Scope
  Scope1 : Scope
  Scope2 : Scope
  Sine Wave : Sin  Frequency=0.05  SampleTime=0
  Square : Math  Operator=square
  Square1 : Math  Operator=square
  Step : Step  Time=0  SampleTime=0
  magTorqueMatrix : Outport
  momentoDipolar : Outport  Port=2
  Mgt_pwr : Outport  Port=3
  wires:
  PID Controller3/1 -> Manual Switch1/2
  Saturation 6V1/1 -> [V1], Scope1/1, MATLAB Function/2(voltageX), Momento Dipolar X/1  "PWR_mgt X"
  Hz_error/1 -> PID Controller2/1, Corrección Y/1("H_error "), Corrección X/1("H_error ")
  Product/1 -> Corrección Y/2(B), Corrección X/2(B), MATLAB Function/1(B), Cross Product2/2, Cross Product1/2, Cross Product/2
  Manual Switch/1 -> Saturation 6V2/1
  PID Controller1/1 -> Manual Switch/1
  Constant/1 -> Manual Switch2/2, MATLAB Function/4(voltageZ), Manual Switch/2
  Constant1/1 -> Manual Switch1/1
  Manual Switch1/1 -> Saturation 6V1/1
  Momento Dipolar X/1 -> Add1/1, Mgt_ejeX/1
  Mgt_ejeX/1 -> Cross Product/1
  Cross Product/1 -> Add/1, Contribucion de cada Mgt/1  "MgtX"
  Saturation 6V2/1 -> [V2], Scope2/1, MATLAB Function/3(voltageY), Momento Dipolar Y/1  "PWR_mgt Y"
  Momento Dipolar Y/1 -> Add1/2, Mgt_ejeY/1
  Mgt_ejeY/1 -> Cross Product1/1
  Cross Product1/1 -> Contribucion de cada Mgt/2, Add/2  "MgtY"
  Add/1 -> Contribucion de cada Mgt1/1, Scope/1, magTorqueMatrix/1
  MATLAB Function/1(magTorqueMatrix) -> Contribucion de cada Mgt1/2
  Add1/1 -> Contribucion de cada Mgt2/1, momentoDipolar/1
  MATLAB Function/2(momentoDipolar) -> Contribucion de cada Mgt2/2
  Manual Switch2/1 -> Saturation 6V3/1
  PID Controller2/1 -> Manual Switch2/1
  Saturation 6V3/1 -> Momento Dipolar Z/1  "PWR_mgt Y"
  Momento Dipolar Z/1 -> Mgt_ejeZ/1
  Mgt_ejeZ/1 -> Cross Product2/1
  Cross Product2/1 -> Add/3  "MgtZ"
  Geomagnetic/1 -> Product/1
  Step/1 -> Product/2
  Corrección X/1(H_error) -> PID Controller3/1
  Corrección Y/1(H_error) -> PID Controller1/1
  Add2/1 -> Mgt_pwr/1
  [V1] -> Square/1
  [V2] -> Square1/1
  Square/1 -> Gain/1
  Square1/1 -> Gain1/1
  Gain/1 -> Add2/1
  Gain1/1 -> Add2/2

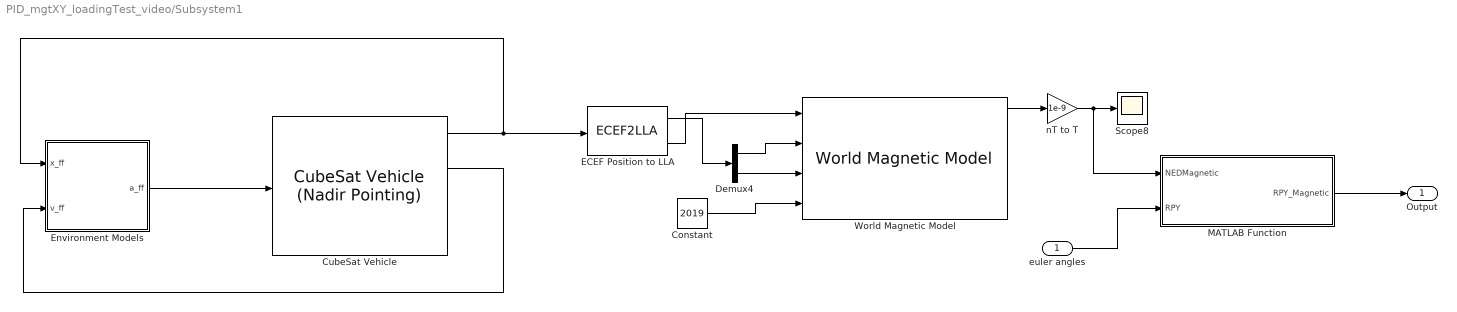
== system PID_mgtXY_loadingTest_video/Subsystem1 ==
  euler angles : Inport
  Constant : Constant  Value=2019
  CubeSat Vehicle : aerolibcubesatveh/CubeSat Vehicle (Nadir Pointing)  sim_t0=juliandate(2019, 1, 4, 12, 0, 0)  method=Keplerian Orbital Elements  epoch=juliandate(2020, 1, 1, 12, 0, 0)  a=6786233.13  ecc=0.0010537  incl=51.7519  omega=95.2562  argp=93.4872  nu=302.9234  truelon=0  arglat=0  lonper=0  r_eci=[0 0 0]  v_eci=[0 0 0]  r_ecef=[0 0 0]  v_ecef=[0 0 0]  lla=[0 0 0]  v_ned=[0 0 0]  euler=[0 0 0]  pqr=[0 0 -0.05168]  pointingMode=Earth (Nadir) Pointing  firstAlignExt=Dialog  firstAlign=[0 0 1]  secondAlignExt=Dialog  secondAlign=[0 1 0]  constraintCoord=ECI Axes  firstRefExt=Dialog  firstRef=[1 0 0]  secondRefExt=Dialog  secondRef=[0 0 1]  missionRTSource=Dialog  missionRT=6*60*60  missionGS=[42, -71]  missionTOICheck=on  missionTOI=[]  missionEta=55
      settings: AttributesFormatString=%<pointingMode>
  Demux4 : Demux  Outputs=2
  ECEF Position to LLA : ECEF2LLA
  Environment Models : Subsystem
      mask Display:
      | port_label('input', 1, 'X_{ECEF}','texmode','on')
      | port_label('input', 2, 'V_{ECEF}','texmode','on')
      | port_label('output', 1, 'A_{ECEF}','texmode','on')
  MATLAB Function : MATLAB Function  TreatAsAtomicUnit=on
  Scope8 : Scope
  World Magnetic Model : aerolibgravity2/World Magnetic Model  model=WMM2015 V2 (2015-2020)  customFile='WMM2020.COF'  units=Metric (MKS)  time_in=on  month=January  day=1  year=2020  action=Error  h_out=on  dec_out=on  inc_out=on  ti_out=on
  nT to T : Gain  Gain=1e-9
  Output : Outport
  wires:
  ECEF Position to LLA/2 -> World Magnetic Model/1
  Environment Models/1(a_ff) -> CubeSat Vehicle/1
  Constant/1 -> World Magnetic Model/4
  nT to T/1 -> MATLAB Function/1(NEDMagnetic), Scope8/1
  World Magnetic Model/1 -> nT to T/1
  CubeSat Vehicle/1 -> ECEF Position to LLA/1, Environment Models/1(x_ff)
  Demux4/2 -> World Magnetic Model/3
  euler angles/1 -> MATLAB Function/2(RPY)
  CubeSat Vehicle/2 -> Environment Models/2(v_ff)
  MATLAB Function/1(RPY_Magnetic) -> Output/1
  ECEF Position to LLA/1 -> Demux4/1
  Demux4/1 -> World Magnetic Model/2

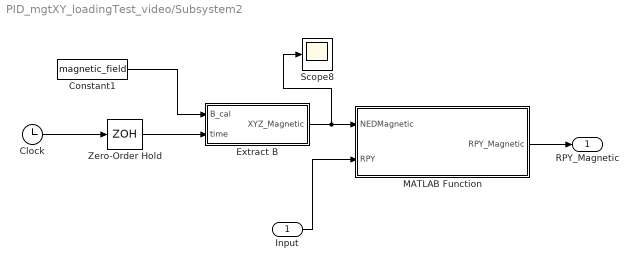
== system PID_mgtXY_loadingTest_video/Subsystem2 ==
  Input : Inport
  Clock : Clock
  Constant1 : Constant  Value=magnetic_field
  Extract B : MATLAB Function  TreatAsAtomicUnit=on
  MATLAB Function : MATLAB Function  TreatAsAtomicUnit=on
  Scope8 : Scope
  Zero-Order Hold : ZeroOrderHold  SampleTime=-1
  RPY_Magnetic : Outport
  wires:
  Constant1/1 -> Extract B/1(B_cal)
  Extract B/1(XYZ_Magnetic) -> MATLAB Function/1(NEDMagnetic), Scope8/1
  Input/1 -> MATLAB Function/2(RPY)
  Zero-Order Hold/1 -> Extract B/2(time)
  MATLAB Function/1(RPY_Magnetic) -> RPY_Magnetic/1
  Clock/1 -> Zero-Order Hold/1

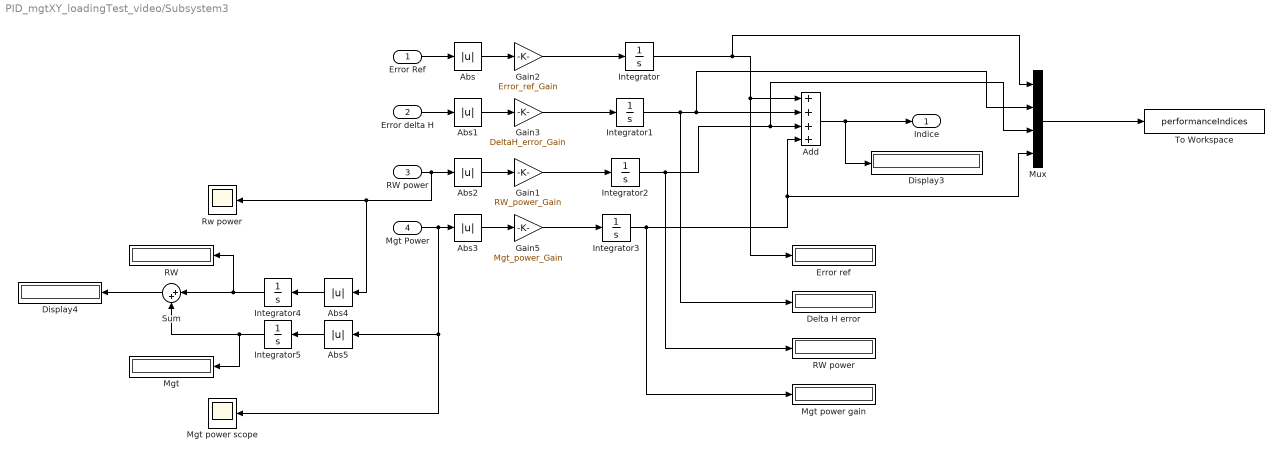
== system PID_mgtXY_loadingTest_video/Subsystem3 ==
  Error Ref : Inport
  Error delta H : Inport  Port=2
  RW power : Inport  Port=3
  Mgt Power : Inport  Port=4
  Abs{,1..5} (6 alike) : Abs  SaturateOnIntegerOverflow=off
  Add : Sum  Inputs=++++
  Delta H error : Display
  Display3 : Display
  Display4 : Display
  Error ref : Display
  Gain1 : Gain  Gain=RW_power_Gain
  Gain2 : Gain  Gain=Error_ref_Gain
  Gain3 : Gain  Gain=DeltaH_error_Gain
  Gain5 : Gain  Gain=Mgt_power_Gain
  Integrator{,1..5} (6 alike) : Integrator
  Mgt : Display
  Mgt power gain : Display
  Mgt power scope : Scope
  Mux : Mux
  RW : Display
  "RW power " : Display
  Rw power : Scope
  Sum : Sum  Inputs=|++
  To Workspace : ToWorkspace  VariableName=performanceIndices  SaveFormat=Structure With Time  SampleTime=-1
  Indice : Outport
  wires:
  Gain1/1 -> Integrator2/1
  Abs1/1 -> Gain3/1
  Abs/1 -> Gain2/1
  Abs2/1 -> Gain1/1
  Abs3/1 -> Gain5/1
  Gain3/1 -> Integrator1/1
  Gain5/1 -> Integrator3/1
  RW power/1 -> Abs4/1, Rw power/1, Abs2/1
  Error delta H/1 -> Abs1/1
  Gain2/1 -> Integrator/1
  Integrator1/1 -> Delta H error/1, Mux/2, Add/2
  Integrator2/1 -> Mux/3, Add/3, "RW power "/1
  Integrator3/1 -> Add/4, Mux/4, Mgt power gain/1
  Add/1 -> Indice/1, Display3/1
  Integrator4/1 -> RW/1, Sum/1
  Integrator5/1 -> Mgt/1, Sum/2
  Sum/1 -> Display4/1
  Mgt Power/1 -> Abs5/1, Mgt power scope/1, Abs3/1
  Abs4/1 -> Integrator4/1
  Abs5/1 -> Integrator5/1
  Error Ref/1 -> Abs/1
  Mux/1 -> To Workspace/1
  Integrator/1 -> Mux/1, Add/1, Error ref/1
